simulink model "Task2"  (R2022a)
settings: Solver=VariableStepAuto  StartTime=0.0  StopTime=10.0  RelTol=1e-3
undefined symbols (not defined in the file): A, A1, Aj, B, B1, Bj, C, C1, Cj
settings Model: Creator=Family  LastModifiedBy=Family

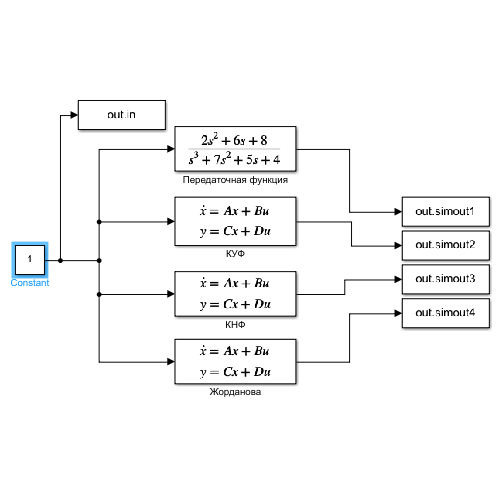
[thumbnail: Simulink's stored preview of the top-level diagram]
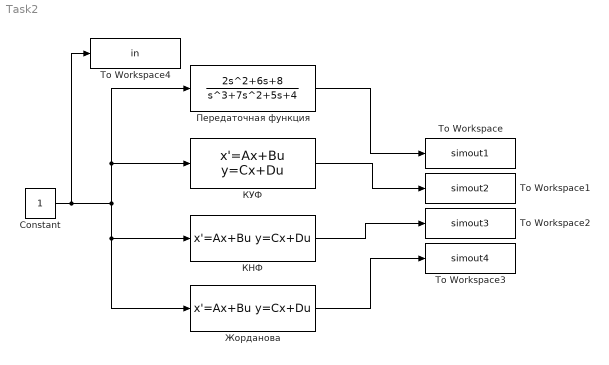
== system Task2 ==
  Constant : Constant  SampleTime=-1
  To Workspace : ToWorkspace  VariableName=simout1  SaveFormat=Timeseries  SampleTime=-1
  To Workspace1 : ToWorkspace  VariableName=simout2  SaveFormat=Timeseries  SampleTime=-1
  To Workspace2 : ToWorkspace  VariableName=simout3  SaveFormat=Timeseries  SampleTime=-1
  To Workspace3 : ToWorkspace  VariableName=simout4  SaveFormat=Timeseries  SampleTime=-1
  To Workspace4 : ToWorkspace  VariableName=in  SaveFormat=Timeseries  SampleTime=-1
  Жорданова : StateSpace  A=Aj  B=Bj  C=Cj  D=0  InitialCondition=0
  КНФ : StateSpace  A=A1  B=B1  C=C1  D=0  InitialCondition=0
  КУФ : StateSpace  A=A  B=B  C=C  D=0  InitialCondition=0
  Передаточная функция : TransferFcn  Numerator=[2 6 8]  Denominator=[1 7 5 4]
  wires:
  Constant/1 -> Передаточная функция/1, КУФ/1, Жорданова/1, КНФ/1, To Workspace4/1
  КУФ/1 -> To Workspace1/1
  Передаточная функция/1 -> To Workspace/1
  КНФ/1 -> To Workspace2/1
  Жорданова/1 -> To Workspace3/1
